simulink model "Lab1_Simulation2025a"  (R2025a)
settings: Solver=VariableStepAuto  StartTime=0.0  StopTime=10000  RelTol=1e-3
values from neighbouring files (symbols this model uses):
  A_num = double(subs(A, [k1 k12 k2 k23 k3], [0.002 0.077 0.004 0.081 0.006]))    [mainTaskLab1.m]    (also in prepareLab1.m = double(subs(A, [R1 R2 R3 C1 C2 C3], [4 4 4 1 1 1])))
  B_num = double(subs(B, [kin], [0.034]))    [mainTaskLab1.m]    (also in prepareLab1.m = double(subs(B, [R1 C1], [4 1])))
  C = [0, 0, 1]    [mainTaskLab1.m]    (also in prepareLab1.m)
  D = 0    [mainTaskLab1.m]    (also in prepareLab1.m)
  F = [kz1   0 ... (first row only)    [mainTaskLab1.m]
settings Model: Creator=Phu  LastModifiedBy=Admin

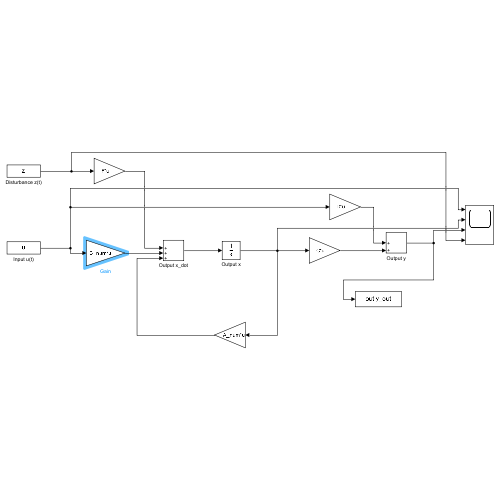
[thumbnail: Simulink's stored preview of the top-level diagram]
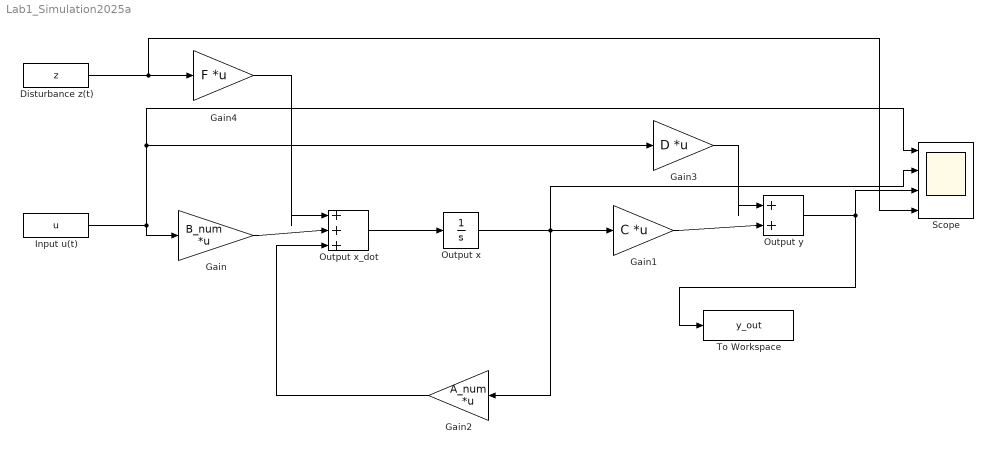
== system Lab1_Simulation2025a ==
  Disturbance z(t) : FromWorkspace  VariableName=z
  Gain : Gain  Gain=B_num  Multiplication=Matrix(K*u)
  Gain1 : Gain  Gain=C  Multiplication=Matrix(K*u)
  Gain2 : Gain  Gain=A_num  Multiplication=Matrix(K*u)
  Gain3 : Gain  Gain=D  Multiplication=Matrix(K*u)
  Gain4 : Gain  Gain=F  Multiplication=Matrix(K*u)
  Input u(t) : FromWorkspace  VariableName=u
  Output x : Integrator
  Output x_dot : Sum  Inputs=|+++
  Output y : Sum  Inputs=|++
  Scope : Scope  NumInputPorts=4
      settings: ActiveDisplayYMinimum=-16.302745367731156  ActiveDisplayYMaximum=86.845170867432714
  To Workspace : ToWorkspace  VariableName=y_out  SaveFormat=Timeseries  SampleTime=-1
  wires:
  Output x_dot/1 -> Output x/1
  Output x/1 -> Scope/2, Gain2/1, Gain1/1
  Output y/1 -> Scope/3, To Workspace/1
  Input u(t)/1 -> Scope/1, Gain3/1, Gain/1
  Disturbance z(t)/1 -> Scope/4, Gain4/1
  Gain3/1 -> Output y/1
  Gain1/1 -> Output y/2
  Gain4/1 -> Output x_dot/1
  Gain/1 -> Output x_dot/2
  Gain2/1 -> Output x_dot/3
